simulink subsystem "hardware"  (R2024a)
settings: Solver=VariableStepAuto  StartTime=0.0  StopTime=10.0  RelTol=1e-3
model mask{RollOffset=0}
  mask prompts: RollOffset "Calibration Roll Offset"
undefined symbols (not defined in the file or in its folder): HS, IO291
libraries: speedgoatlib_IO691 x12, canmsglib x9, eeGeneralControl x6, aru_toolbox x4, speedgoatlib_IO291 x1
settings Model: Creator=Mechatronics  LastModifiedBy=user
settings ModelReferenceCC: EnableRefExpFcnMdlSchedulingChecks=on
settings RTWCC: GPUComputeCapability=3.5

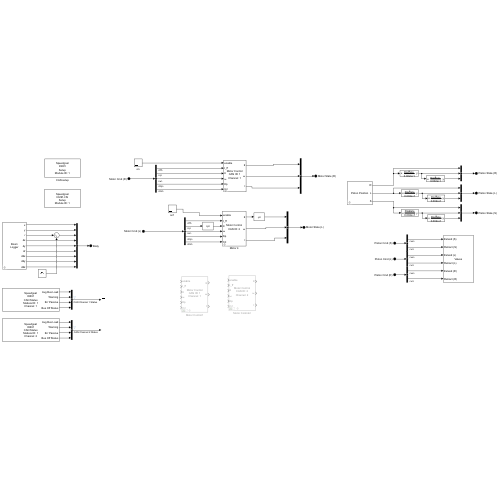
[thumbnail: Simulink's stored preview of the top-level diagram]
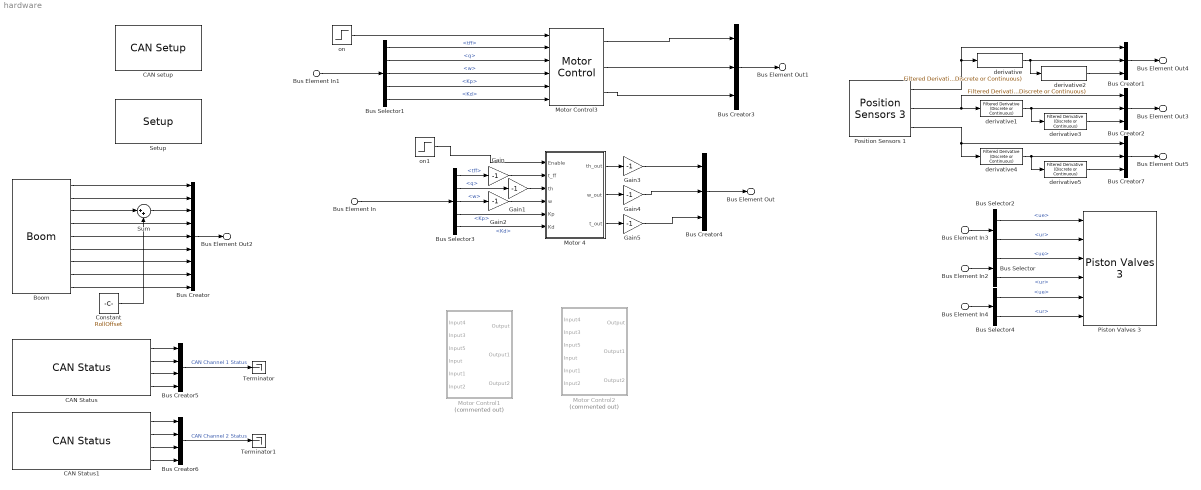
== system hardware ==
  Bus Element In : Inport  PortName=Motor Cmd (R)
  Bus Element In4 : Inport  Port=2  PortName=Piston Cmd (R)
  Bus Element In1 : Inport  Port=3  PortName=Motor Cmd (L)
  Bus Element In2 : Inport  Port=4  PortName=Piston Cmd (L)
  Bus Element In3 : Inport  Port=5  PortName=Piston Cmd (S)
  Boom : aru_toolbox/Boom  ts=0.001
      link override Serial Read HW FIFO: pciSlot=-1  board=IO393-50k
      link override Serial Setup: pciSlot=-1  board=IO393-50k
      settings: SourceProductName=ARU Toolbox
  Bus Creator : BusCreator  Inputs=9  OutDataTypeStr=Bus: BodyState  NonVirtualBus=on
      settings: InheritFromInputs=off
  Bus Creator1 : BusCreator  Inputs=3  OutDataTypeStr=Bus: PistonState  NonVirtualBus=on
      settings: InheritFromInputs=off
  Bus Creator2 : BusCreator  Inputs=3  OutDataTypeStr=Bus: PistonState  NonVirtualBus=on
      settings: InheritFromInputs=off
  Bus Creator3 : BusCreator  Inputs=3  OutDataTypeStr=Bus: MotorState  NonVirtualBus=on
      settings: InheritFromInputs=off
  Bus Creator4 : BusCreator  Inputs=3  OutDataTypeStr=Bus: MotorState  NonVirtualBus=on
      settings: InheritFromInputs=off
  Bus Creator5 : BusCreator  Inputs=4  OutDataTypeStr=Bus: CAN  NonVirtualBus=on
      settings: InheritFromInputs=off
  Bus Creator6 : BusCreator  Inputs=4  OutDataTypeStr=Bus: CAN  NonVirtualBus=on
      settings: InheritFromInputs=off
  Bus Creator7 : BusCreator  Inputs=3  OutDataTypeStr=Bus: PistonState  NonVirtualBus=on
      settings: InheritFromInputs=off
  Bus Selector : BusSelector  OutputSignals=ue,ur
  Bus Selector1 : BusSelector  OutputSignals=tff,q,w,Kp,Kd
  Bus Selector2 : BusSelector  OutputSignals=ue,ur
  Bus Selector3 : BusSelector  OutputSignals=tff,q,w,Kp,Kd
  Bus Selector4 : BusSelector  OutputSignals=ue,ur
  CAN Status : speedgoatlib_IO691/Legacy/CAN Status  moduleId=1  sampleTime=0.001  channel=1  busRecovery=Auto  arrayOutput=off  controllerCpuLoad=off  controllerLiveCount=off  initModeAct=off  avgBusLoad=on  receiving=off  RxQueueEmpty=off  dataOverrunRcv=off  rxBufferLevel=off  txPending=off  dataOverrunTx=off  txBufferLevel=off  errWarnLimit=on  errPassLimit=on  errBusOff=on  busRecoveryCounter=off  busCouplingErr=off  transceiverErr=off  opMode=off  brp=off  timeSegment1=off  timeSegment2=off  synchronisationJumpWidth=off  dataTSEG1=off  dataTSEG2=off  dataSJW=off  moduleType=691  qtyStatBlk=1  ptIdx=0  isFDMod=0
      settings: SourceProductName=IO691
  CAN Status1 : speedgoatlib_IO691/Legacy/CAN Status  moduleId=1  sampleTime=0.001  channel=2  busRecovery=Auto  arrayOutput=off  controllerCpuLoad=off  controllerLiveCount=off  initModeAct=off  avgBusLoad=on  receiving=off  RxQueueEmpty=off  dataOverrunRcv=off  rxBufferLevel=off  txPending=off  dataOverrunTx=off  txBufferLevel=off  errWarnLimit=on  errPassLimit=on  errBusOff=on  busRecoveryCounter=off  busCouplingErr=off  transceiverErr=off  opMode=off  brp=off  timeSegment1=off  timeSegment2=off  synchronisationJumpWidth=off  dataTSEG1=off  dataTSEG2=off  dataSJW=off  moduleType=691  qtyStatBlk=1  ptIdx=0  isFDMod=0
      settings: SourceProductName=IO691
  CAN setup : speedgoatlib_IO691/Legacy/CAN Setup   moduletype=IO691  id=1  pciSlot=-1  chn1=CAN (HS)  chn2=CAN (HS)  chn3=Disabled  chn4=Disabled  initStruct=[]  termStruct=[struct('Channel',1,'Protocol','CAN','BRS',0,'Type','Standard','Identifier',1,'Data',[255, 255, 255, 255, 255, 255, 255, 253],'Pause',0.001), struct('Channel',2,'Protocol','CAN','BRS',0,'Type','Standard','Identifier',2,'Data',[255, 255, 255, 255, 255, 255, 255, 253],'Pause',0.001)]  ArbitrationbdrChn1=1.0 MBaud  ArbitrationManbdrChn1=[2,8,31,8]  FdbdrChn1=1.0 MBaud  FdManbdrChn1=[2,8,31,8]  ArbitrationbdrChn2=1.0 MBaud  ArbitrationManbdrChn2=[2,8,31,8]  FdbdrChn2=1.0 MBaud  FdManbdrChn2=[2,8,31,8]  ArbitrationbdrChn3=1.0 MBaud  ArbitrationManbdrChn3=[2,8,31,8]  FdbdrChn3=5.0 MBaud  FdManbdrChn3=[2,2,5,2]  ArbitrationbdrChn4=1.0 MBaud  ArbitrationManbdrChn4=[2,8,31,8]  FdbdrChn4=5.0 MBaud  FdManbdrChn4=[2,2,5,2]  moduleInitValues=[691 1 -1 -1]
      settings: SourceProductName=IO691
  Constant : Constant  Value=RollOffset
  Gain{,1..5} (6 alike) : Gain  Gain=-1
  Motor 4 : Subsystem  mask{CAN_ID=2, channel=1}
      mask prompts: CAN_ID "CAN ID"
      mask init:
      | if exist("CAN_ID", "var")
      |         if CAN_ID == 1
      |             channel = 1;
      |             % set_param([gcb '/Enter Motor Mode/CAN Write Command'],'channel',sprintf('%d',1));
      |             % set_param([gcb '/CAN Write/CAN Write Command'],'channel',sprintf('%d',1));
      |             % set_param([gcb '/CAN Read/CAN Read Command'],'channel',sprintf('%d',1));
      |         end
      |         if CAN_ID == 2
      |             channel = 2;
      |             % set_param([gcb '/Enter Motor Mode/CAN Write Command'],'channel',sprintf('%d',2));
      |             % set_param([gcb '/CAN Write/CAN Write Command'],'channel',sprintf('%d',2));
      |             % set_param([gcb '/CAN Read/CAN Read Command'],'channel',sprintf('%d',2));
      |         end
      |     end
      mask TypeOptions channel: 1 | 2
      mask Display:
      | fprintf('Motor Control\nCAN ID: %c\n', get_param(gcb,'CAN_ID'));
      | port_label('input',1,'enable');
      | port_label('input',2,'t_ff');
      | port_label('input',3,'θ');
      | port_label('input',4,'ω');
      | port_label('input',5,'Kp');
      | port_label('input',6,'Kd');
      | port_label('output',1,'θ');
      | port_label('output',2,'ω');
      | port_label('output',3,'t');
  Motor Control1 : Subsystem  Commented=on  AncestorBlock=aru_toolbox/Motor Control  mask(Motor Control){id=1, channel=1, offset=-pi}
      mask prompts: offset "Position Offset (rad)"
      mask help: Generic control block for motors running Ben Katz's motor control firmware. (https://github.com/bgkatz/motorcontrol)
      mask TypeOptions channel: 1 | 2
      mask DialogControl ParameterGroupVar Prompt: CAN
      mask DialogControl Container4 Prompt: Control
      mask Display:
      | fprintf('Motor Control\nCAN ID: %c\nChannel: %c\n', get_param(gcb,'id'), get_param(gcb,'channel'));
      | port_label('input',1,'enable');
      | port_label('input',2,'t_ff');
      | port_label('input',3,'θ');
      | port_label('input',4,'ω');
      | port_label('input',5,'Kp');
      | port_label('input',6,'Kd');
      | port_label('output',1,'θ');
      | port_label('output',2,'ω');
      | port_label('output',3,'t');
  Motor Control2 : Subsystem  Commented=on  AncestorBlock=aru_toolbox/Motor Control  mask(Motor Control){id=2, channel=2, offset=0}
      mask prompts: offset "Position Offset (rad)"
      mask help: Generic control block for motors running Ben Katz's motor control firmware. (https://github.com/bgkatz/motorcontrol)
      mask TypeOptions channel: 1 | 2
      mask DialogControl ParameterGroupVar Prompt: CAN
      mask DialogControl Container4 Prompt: Control
      mask Display:
      | fprintf('Motor Control\nCAN ID: %c\nChannel: %c\n', get_param(gcb,'id'), get_param(gcb,'channel'));
      | port_label('input',1,'enable');
      | port_label('input',2,'t_ff');
      | port_label('input',3,'θ');
      | port_label('input',4,'ω');
      | port_label('input',5,'Kp');
      | port_label('input',6,'Kd');
      | port_label('output',1,'θ');
      | port_label('output',2,'ω');
      | port_label('output',3,'t');
  Motor Control3 : aru_toolbox/Motor Control  id=1  channel=1  offset=0
      settings: SourceProductName=ARU Toolbox
  Piston Valves 3 : aru_toolbox/Piston Valves 3  SystemSampleTime=-1  VariantActivationTime=update diagram  AllowFlexibleInterface=on  Latency=0  AutoFrameSizeCalculation=off
      settings: SourceProductName=ARU Toolbox
  Position Sensors 1 : aru_toolbox/Position Sensors 3  stroke1=0.07  min_r=803  max_r=3724  stroke2=0.07  min_l=743  max_l=3646  stroke3=0.2  min_s=741  max_s=3392
      settings: SourceProductName=ARU Toolbox
  "Setup " : speedgoatlib_IO291/Setup   parInternalModuleId=1  parPciSlot=-1  parModuleId=1  parModuleType=IO291-HS  parTtlDoChannels=[]  parTtlDoInitValues=1  parTtlDoReset=1  parTtlDiChannels=[1 2 3 4 5]  parIsolDiChannels=[]  parFetDoChannels=[1 2 3 4 5 6]  parFetDoInitValues=0  parFetDoReset=1
      settings: SourceProductName=IO291
  Sum : Sum  Inputs=|++
  Terminator : Terminator
  Terminator1 : Terminator
  derivative{,1..5} (6 alike) : eeGeneralControl/Filtered Derivative (Discrete or Continuous)  K=1  T=0.002  B=inf  A=-inf  minRatio=2  init_option=Inherited from block input  x0=0  Ts=0.001
  on : Step  SampleTime=0
  on1 : Step  Time=2  SampleTime=0
  Bus Element Out : Outport  PortName=Motor State (R)
  Bus Element Out4 : Outport  Port=2  PortName=Piston State (R)
  Bus Element Out1 : Outport  Port=3  PortName=Motor State (L)
  Bus Element Out3 : Outport  Port=4  PortName=Piston State (L)
  Bus Element Out2 : Outport  Port=5  PortName=Body
  Bus Element Out5 : Outport  Port=6  PortName=Piston State (S)
  wires:
  Bus Selector1/1 -> Motor Control3/2  "<tff>"
  Bus Creator5/1 -> Terminator/1  "CAN Channel 1 Status"
  derivative2/1 -> Bus Creator1/3
  Bus Selector/1 -> Piston Valves 3/3  "<ue>"
  Bus Element In1/1 -> Bus Selector1/1
  Bus Selector1/4 -> Motor Control3/5  "<Kp>"
  Bus Selector/2 -> Piston Valves 3/4  "<ur>"
  Bus Selector3/4 -> Motor 4/5(Kp)  "<Kp>"
  Bus Selector3/2 -> Gain1/1  "<q>"
  Bus Selector2/2 -> Piston Valves 3/2  "<ur>"
  Bus Creator6/1 -> Terminator1/1  "CAN Channel 2 Status"
  CAN Status1/3 -> Bus Creator6/3
  on1/1 -> Motor 4/1(Enable)
  Bus Selector2/1 -> Piston Valves 3/1  "<ue>"
  Bus Element In3/1 -> Bus Selector2/1
  Bus Selector1/3 -> Motor Control3/4  "<w>"
  CAN Status1/4 -> Bus Creator6/4
  Bus Selector3/1 -> Gain/1  "<tff>"
  Boom/1 -> Bus Creator/1
  Boom/3 -> Sum/1
  Bus Element In2/1 -> Bus Selector/1
  CAN Status/3 -> Bus Creator5/3
  Bus Creator1/1 -> Bus Element Out4/1
  Boom/7 -> Bus Creator/7
  Boom/5 -> Bus Creator/5
  Boom/6 -> Bus Creator/6
  Bus Creator/1 -> Bus Element Out2/1
  Bus Selector3/5 -> Motor 4/6(Kd)  "<Kd>"
  Boom/8 -> Bus Creator/8
  Boom/4 -> Bus Creator/4
  Bus Selector1/2 -> Motor Control3/3  "<q>"
  derivative/1 -> derivative2/1, Bus Creator1/2
  derivative3/1 -> Bus Creator2/3
  CAN Status/4 -> Bus Creator5/4
  Bus Selector3/3 -> Gain2/1  "<w>"
  derivative1/1 -> derivative3/1, Bus Creator2/2
  Boom/2 -> Bus Creator/2
  CAN Status1/2 -> Bus Creator6/2
  Position Sensors 1/2 -> derivative1/1, Bus Creator2/1
  Bus Element In/1 -> Bus Selector3/1
  Bus Selector1/5 -> Motor Control3/6  "<Kd>"
  Constant/1 -> Sum/2
  CAN Status/1 -> Bus Creator5/1
  Boom/9 -> Bus Creator/9
  Position Sensors 1/1 -> Bus Creator1/1, derivative/1
  Sum/1 -> Bus Creator/3
  on/1 -> Motor Control3/1
  CAN Status1/1 -> Bus Creator6/1
  Bus Creator2/1 -> Bus Element Out3/1
  CAN Status/2 -> Bus Creator5/2
  Motor 4/2(w_out) -> Gain4/1
  Motor 4/3(t_out) -> Gain5/1
  Bus Selector4/2 -> Piston Valves 3/6  "<ur>"
  Bus Selector4/1 -> Piston Valves 3/5  "<ue>"
  Bus Element In4/1 -> Bus Selector4/1
  derivative4/1 -> derivative5/1, Bus Creator7/2
  Bus Creator7/1 -> Bus Element Out5/1
  derivative5/1 -> Bus Creator7/3
  Position Sensors 1/3 -> Bus Creator7/1, derivative4/1
  Motor Control3/1 -> Bus Creator3/1
  Motor Control3/2 -> Bus Creator3/2
  Motor Control3/3 -> Bus Creator3/3
  Motor 4/1(th_out) -> Gain3/1
  Bus Creator4/1 -> Bus Element Out/1
  Bus Creator3/1 -> Bus Element Out1/1
  Gain/1 -> Motor 4/2(t_ff)
  Gain1/1 -> Motor 4/3(th)
  Gain2/1 -> Motor 4/4(w)
  Gain3/1 -> Bus Creator4/1
  Gain4/1 -> Bus Creator4/2
  Gain5/1 -> Bus Creator4/3

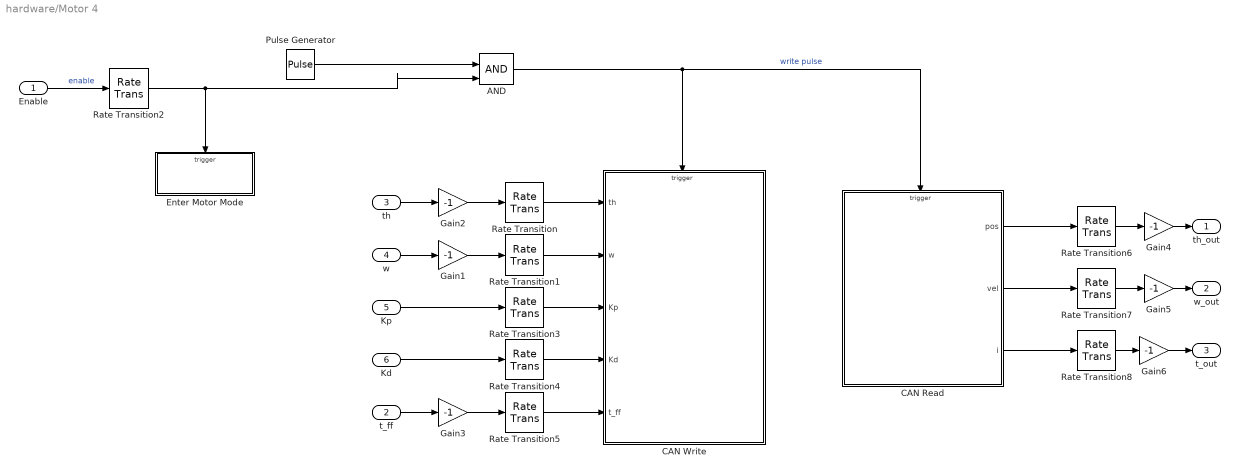
== system hardware/Motor 4 ==
  Enable : Inport
  t_ff : Inport  Port=2
  th : Inport  Port=3
  w : Inport  Port=4
  Kp : Inport  Port=5
  Kd : Inport  Port=6
  AND : Logic  IconShape=distinctive  AllPortsSameDT=off  OutDataTypeStr=boolean
  CAN Read : Subsystem  LoadFcn=set_param([gcb '/CAN Read Command'], 'channel', sprintf('%d', channel));  TreatAsAtomicUnit=on
  CAN Write : Subsystem  LoadFcn=set_param([gcb '/CAN Write Command'], 'channel', sprintf('%d', channel));
  Enter Motor Mode : Subsystem  LoadFcn=set_param([gcb '/CAN Write Command'], 'channel', sprintf('%d', channel));  TreatAsAtomicUnit=on
  Gain{1..6} (6 alike) : Gain  Gain=-1
  Pulse Generator : DiscretePulseGenerator  PulseType=Time based  Period=1/1000  PulseWidth=50
  Rate Transition{,1..8} (9 alike) : RateTransition
  th_out : Outport
  w_out : Outport  Port=2
  t_out : Outport  Port=3
  wires:
  Gain6/1 -> t_out/1
  Gain5/1 -> w_out/1
  Gain4/1 -> th_out/1
  Gain3/1 -> Rate Transition5/1
  Gain1/1 -> Rate Transition1/1
  Gain2/1 -> Rate Transition/1
  Rate Transition2/1 -> Enter Motor Mode/Trigger, AND/2
  Pulse Generator/1 -> AND/1
  AND/1 -> CAN Read/Trigger, CAN Write/Trigger  "write pulse"
  Enable/1 -> Rate Transition2/1  "enable"
  Rate Transition5/1 -> CAN Write/5(t_ff)
  Rate Transition/1 -> CAN Write/1(th)
  th/1 -> Gain2/1
  t_ff/1 -> Gain3/1
  Kd/1 -> Rate Transition4/1
  Kp/1 -> Rate Transition3/1
  w/1 -> Gain1/1
  Rate Transition1/1 -> CAN Write/2(w)
  Rate Transition3/1 -> CAN Write/3(Kp)
  Rate Transition4/1 -> CAN Write/4(Kd)
  CAN Read/1(pos) -> Rate Transition6/1
  CAN Read/2(vel) -> Rate Transition7/1
  CAN Read/3(i) -> Rate Transition8/1
  Rate Transition6/1 -> Gain4/1
  Rate Transition8/1 -> Gain6/1
  Rate Transition7/1 -> Gain5/1

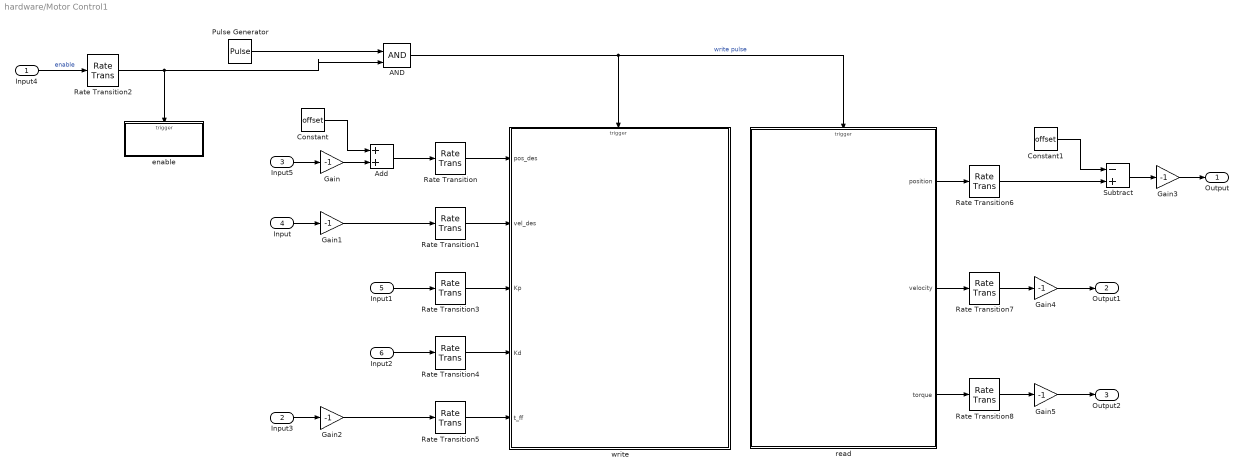
== system hardware/Motor Control1 ==
  Input4 : Inport
  Input3 : Inport  Port=2
  Input5 : Inport  Port=3
  Input : Inport  Port=4
  Input1 : Inport  Port=5
  Input2 : Inport  Port=6
  AND : Logic  IconShape=distinctive  AllPortsSameDT=off  OutDataTypeStr=boolean
  Add : Sum
  Constant : Constant  Value=offset
  Constant1 : Constant  Value=offset
  Gain{,1..5} (6 alike) : Gain  Gain=-1
  Pulse Generator : DiscretePulseGenerator  PulseType=Time based  Period=0.001  PulseWidth=50
  Rate Transition{,1..8} (9 alike) : RateTransition
  Subtract : Sum  Inputs=-+
  enable : Subsystem  TreatAsAtomicUnit=on
  read : Subsystem  TreatAsAtomicUnit=on
  write : Subsystem  TreatAsAtomicUnit=on
  Output : Outport
  Output1 : Outport  Port=2
  Output2 : Outport  Port=3
  wires:
  Gain5/1 -> Output2/1
  Gain4/1 -> Output1/1
  Gain3/1 -> Output/1
  Gain2/1 -> Rate Transition5/1
  Gain1/1 -> Rate Transition1/1
  Gain/1 -> Add/2
  Constant1/1 -> Subtract/1
  Rate Transition6/1 -> Subtract/2
  Subtract/1 -> Gain3/1
  Constant/1 -> Add/1
  Add/1 -> Rate Transition/1
  Input5/1 -> Gain/1
  Rate Transition8/1 -> Gain5/1
  Rate Transition7/1 -> Gain4/1
  Rate Transition5/1 -> write/5(t_ff)
  Rate Transition4/1 -> write/4(Kd)
  Rate Transition3/1 -> write/3(Kp)
  Rate Transition2/1 -> AND/2, enable/Trigger
  Rate Transition1/1 -> write/2(vel_des)
  Rate Transition/1 -> write/1(pos_des)
  read/1(position) -> Rate Transition6/1
  Input4/1 -> Rate Transition2/1  "enable"
  AND/1 -> write/Trigger, read/Trigger  "write pulse"
  Pulse Generator/1 -> AND/1
  Input/1 -> Gain1/1
  read/3(torque) -> Rate Transition8/1
  read/2(velocity) -> Rate Transition7/1
  Input2/1 -> Rate Transition4/1
  Input3/1 -> Gain2/1
  Input1/1 -> Rate Transition3/1

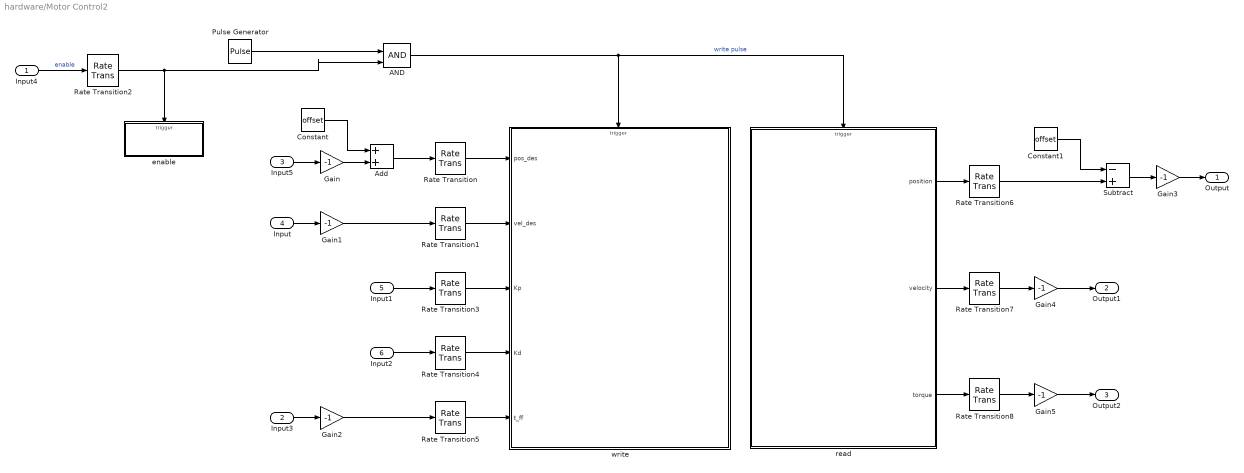
== system hardware/Motor Control2 ==
  Input4 : Inport
  Input3 : Inport  Port=2
  Input5 : Inport  Port=3
  Input : Inport  Port=4
  Input1 : Inport  Port=5
  Input2 : Inport  Port=6
  AND : Logic  IconShape=distinctive  AllPortsSameDT=off  OutDataTypeStr=boolean
  Add : Sum
  Constant : Constant  Value=offset
  Constant1 : Constant  Value=offset
  Gain{,1..5} (6 alike) : Gain  Gain=-1
  Pulse Generator : DiscretePulseGenerator  PulseType=Time based  Period=0.001  PulseWidth=50
  Rate Transition{,1..8} (9 alike) : RateTransition
  Subtract : Sum  Inputs=-+
  enable : Subsystem  TreatAsAtomicUnit=on
  read : Subsystem  TreatAsAtomicUnit=on
  write : Subsystem  TreatAsAtomicUnit=on
  Output : Outport
  Output1 : Outport  Port=2
  Output2 : Outport  Port=3
  wires:
  Input1/1 -> Rate Transition3/1
  Input3/1 -> Gain2/1
  Input2/1 -> Rate Transition4/1
  read/2(velocity) -> Rate Transition7/1
  read/3(torque) -> Rate Transition8/1
  Input/1 -> Gain1/1
  Pulse Generator/1 -> AND/1
  AND/1 -> read/Trigger, write/Trigger  "write pulse"
  Input4/1 -> Rate Transition2/1  "enable"
  read/1(position) -> Rate Transition6/1
  Rate Transition/1 -> write/1(pos_des)
  Rate Transition1/1 -> write/2(vel_des)
  Rate Transition2/1 -> enable/Trigger, AND/2
  Rate Transition3/1 -> write/3(Kp)
  Rate Transition4/1 -> write/4(Kd)
  Rate Transition5/1 -> write/5(t_ff)
  Rate Transition7/1 -> Gain4/1
  Rate Transition8/1 -> Gain5/1
  Input5/1 -> Gain/1
  Add/1 -> Rate Transition/1
  Constant/1 -> Add/1
  Subtract/1 -> Gain3/1
  Rate Transition6/1 -> Subtract/2
  Constant1/1 -> Subtract/1
  Gain/1 -> Add/2
  Gain1/1 -> Rate Transition1/1
  Gain2/1 -> Rate Transition5/1
  Gain3/1 -> Output/1
  Gain4/1 -> Output1/1
  Gain5/1 -> Output2/1

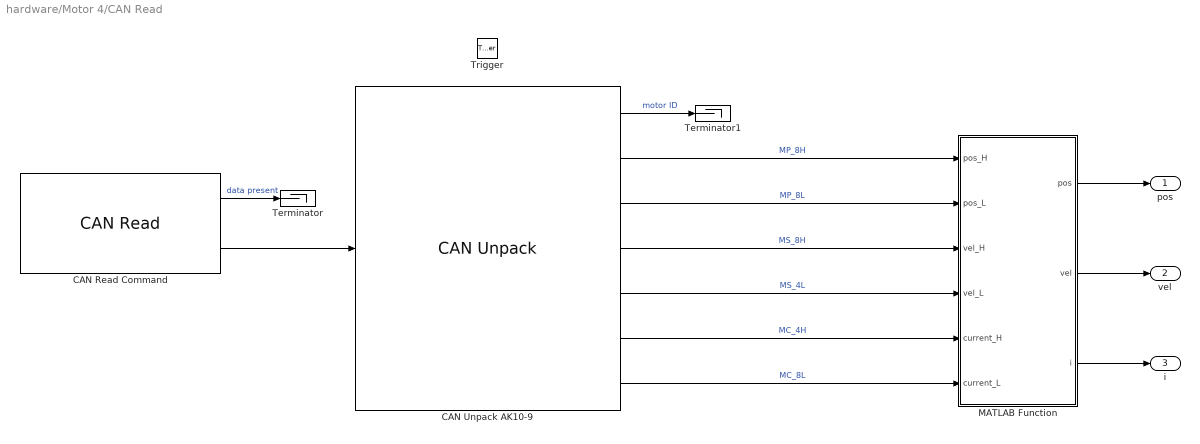
== system hardware/Motor 4/CAN Read ==
  Trigger : TriggerPort  TriggerType=either  VariantControl=(inherit)  PortDimensions=1
  CAN Read Command : speedgoatlib_IO691/Legacy/CAN Read  id=1  ts=-1  channel=2  messageType=CAN  canType=CAN (HS)  BusOutput=off  initValues=[691 1 -1 1 1 1 0]
      settings: SourceProductName=IO691
  CAN Unpack AK10-9 : canmsglib/CAN Unpack  MsgList=(none)  MsgName=CAN Msg  MsgIDType=Standard (11-bit identifier)  MsgIdentifier=0  MsgLength=8  SignalInfo={ 'Drive ID', '0', '8', 'LE', 'unsigned', 'Standard', '0', '1', '0', '-Inf', 'Inf'; 'Motor position 8-H', '8', '8', 'LE', 'unsigned', 'Standard', '0', '1', '0', '-Inf', 'Inf'; 'Motor position 8-L', '16', '8', 'LE', 'unsigned', 'Standard', '0', '1', '0', '-Inf', 'Inf'; 'Motor speed 8-H', '24', '8', 'LE', 'unsigned', 'Standard', '0', '1', '0', '-Inf', 'Inf'; 'Motor speed 4-L', '36', '4', 'LE', 'unsigned', 'Standard', '0', '1', '0', '-Inf', 'Inf'; 'Current 4-H', '32', '4', 'LE', 'unsigned', 'Standard', '0', '1', '0', '-Inf', 'Inf'; 'Current 8-L', '40', '8', 'LE', 'unsigned', 'Standard', '0', '1', '0', '-Inf', 'Inf' }  IDPort=off  TimestampPort=off  ErrorPort=off  RemotePort=off  LengthPort=off  StatusPort=off  ApplyMinMax=off
  MATLAB Function : MATLAB Function  TreatAsAtomicUnit=on
  Terminator : Terminator
  Terminator1 : Terminator
  pos : Outport
  vel : Outport  Port=2
  i : Outport  Port=3
  wires:
  CAN Unpack AK10-9/4 -> MATLAB Function/3(vel_H)  "MS_8H"
  MATLAB Function/1(pos) -> pos/1
  CAN Unpack AK10-9/7 -> MATLAB Function/6(current_L)  "MC_8L"
  CAN Unpack AK10-9/6 -> MATLAB Function/5(current_H)  "MC_4H"
  CAN Unpack AK10-9/2 -> MATLAB Function/1(pos_H)  "MP_8H"
  CAN Unpack AK10-9/1 -> Terminator1/1  "motor ID"
  CAN Unpack AK10-9/5 -> MATLAB Function/4(vel_L)  "MS_4L"
  CAN Unpack AK10-9/3 -> MATLAB Function/2(pos_L)  "MP_8L"
  MATLAB Function/3(i) -> i/1
  MATLAB Function/2(vel) -> vel/1
  CAN Read Command/1 -> Terminator/1  "data present"
  CAN Read Command/2 -> CAN Unpack AK10-9/1

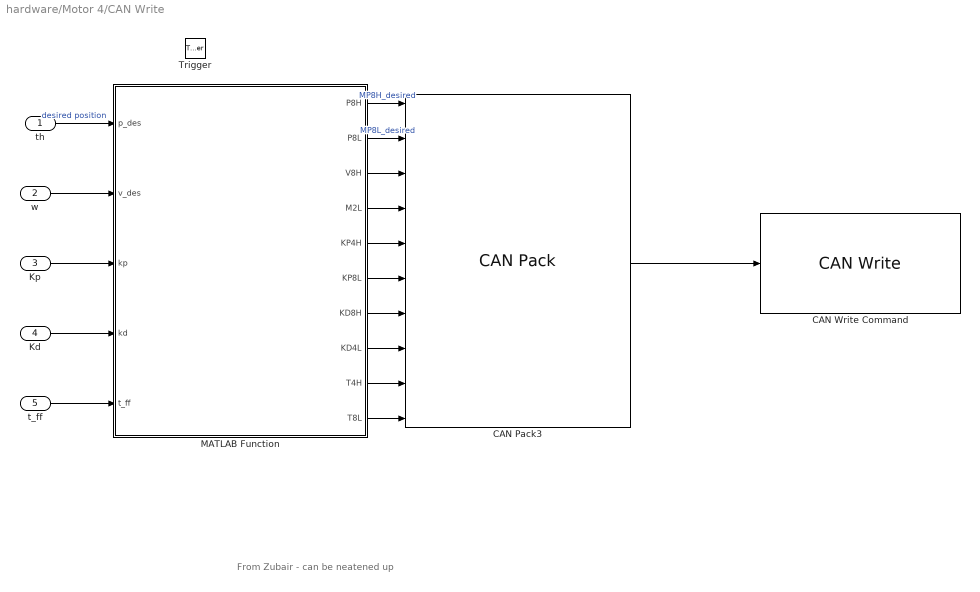
== system hardware/Motor 4/CAN Write ==
  note: From Zubair - can be neatened up
  th : Inport
  w : Inport  Port=2
  Kp : Inport  Port=3
  Kd : Inport  Port=4
  t_ff : Inport  Port=5
  Trigger : TriggerPort  VariantControl=Variant
  CAN Pack3 : canmsglib/CAN Pack  MsgList=(none)  MsgName=MotorControl  MsgIDType=Standard (11-bit identifier)  MsgIdentifier=CAN_ID  MsgLength=8  Remote=off  ApplyMinMax=off  BusOutput=off  SignalInfo={ 'Motor postition 8-H', '0', '8', 'LE', 'unsigned', 'Standard', '0', '1', '0', '-Inf', 'Inf'; 'Motor position 8-L', '8', '8', 'LE', 'unsigned', 'Standard', '0', '1', '0', '-Inf', 'Inf'; 'Motor speed 8-H', '16', '8', 'LE', 'unsigned', 'Standard', '0', '1', '0', '-Inf', 'Inf'; 'Motor speed 4-L', '28', '4', 'LE', 'unsigned', 'Standard', '0', '1', '0', '-Inf', 'Inf'; 'KP 4-H', '24', '4', 'LE', 'unsigned', 'Standard', '0', '1', '0', '-Inf', 'Inf'; 'KP 8-L', '32', '8', 'LE', 'unsigned', 'Standard', '0', '1', '0', '-Inf', 'Inf'; 'KD 8-H', '40', '8', 'LE', 'unsigned', 'Standard', '0', '1', '0', '-Inf', 'Inf'; 'KD 4-L', '52', '4', 'LE', 'unsigned', 'Standard', '0', '1', '0', '-Inf', 'Inf'; 'Current 4-H', '48', '4', 'LE', 'unsigned', 'Standard', '0', '1', '0', '-Inf', 'Inf'; 'Current 8-L', '56', '8', 'LE', 'unsigned', 'Standard', '0', '1', '0', '-Inf', 'Inf' }
      settings: DataFormat=manually specified signals
  CAN Write Command : speedgoatlib_IO691/Legacy/CAN Write  id=1  ts=-1  channel=2  messageType=CAN  BusInput=off  enableStatusPort=off  canType=CAN (HS)  initValues=[691 1 -1 1 1 1 0 0]
      settings: SourceProductName=IO691
  MATLAB Function : MATLAB Function  TreatAsAtomicUnit=on
  wires:
  CAN Pack3/1 -> CAN Write Command/1
  MATLAB Function/1(P8H) -> CAN Pack3/1  "MP8H_desired"
  MATLAB Function/7(KD8H) -> CAN Pack3/7
  Kp/1 -> MATLAB Function/3(kp)
  MATLAB Function/9(T4H) -> CAN Pack3/9
  w/1 -> MATLAB Function/2(v_des)
  Kd/1 -> MATLAB Function/4(kd)
  MATLAB Function/6(KP8L) -> CAN Pack3/6
  th/1 -> MATLAB Function/1(p_des)  "desired position"
  MATLAB Function/10(T8L) -> CAN Pack3/10
  MATLAB Function/2(P8L) -> CAN Pack3/2  "MP8L_desired"
  MATLAB Function/5(KP4H) -> CAN Pack3/5
  MATLAB Function/3(V8H) -> CAN Pack3/3
  t_ff/1 -> MATLAB Function/5(t_ff)
  MATLAB Function/8(KD4L) -> CAN Pack3/8
  MATLAB Function/4(M2L) -> CAN Pack3/4

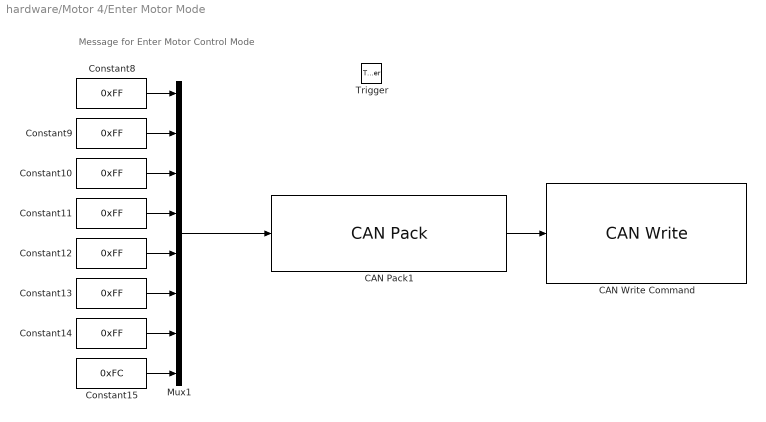
== system hardware/Motor 4/Enter Motor Mode ==
  note: Message for Enter Motor Control Mode
  Trigger : TriggerPort  VariantControl=(inherit)
  CAN Pack1 : canmsglib/CAN Pack  MsgList=(none)  MsgName=CAN Msg  MsgIDType=Standard (11-bit identifier)  MsgIdentifier=CAN_ID  MsgLength=8  Remote=off  ApplyMinMax=off  BusOutput=off  SignalInfo={ 'Motor postition 8-H', '0', '8', 'LE', 'unsigned', 'Standard', '0', '1', '0', '-Inf', 'Inf'; 'Motor position 8-L', '8', '8', 'LE', 'unsigned', 'Standard', '0', '1', '0', '-Inf', 'Inf'; 'Motor seed 8-H', '16', '8', 'LE', 'unsigned', 'Standard', '0', '1', '0', '-Inf', 'Inf'; 'Motor speed 4-L', '28', '4', 'LE', 'unsigned', 'Standard', '0', '1', '0', '-Inf', 'Inf'; 'KP 4-H', '24', '4', 'LE', 'unsigned', 'Standard', '0', '1', '0', '-Inf', 'Inf'; 'KP 8-L', '32', '8', 'LE', 'unsigned', 'Standard', '0', '1', '0', '-Inf', 'Inf'; 'KP 8-H', '40', '8', 'LE', 'unsigned', 'Standard', '0', '1', '0', '-Inf', 'Inf'; 'KD 4-L', '52', '4', 'LE', 'unsigned', 'Standard', '0', '1', '0', '-Inf', 'Inf'; 'Current 4-H', '48', '4', 'LE', 'unsigned', 'Standard', '0', '1', '0', '-Inf', 'Inf'; 'Current 8-L', '56', '8', 'LE', 'unsigned', 'Standard', '0', '1', '0', '-Inf', 'Inf' }
      settings: DataFormat=raw data
  CAN Write Command : speedgoatlib_IO691/Legacy/CAN Write  id=1  ts=-1  channel=2  messageType=CAN  BusInput=off  enableStatusPort=off  canType=CAN (HS)  initValues=[691 1 -1 1 1 1 0 0]
      settings: SourceProductName=IO691
  Constant{8..14} (7 alike) : Constant  Value=0xFF  OutDataTypeStr=uint8  SampleTime=-1
  Constant15 : Constant  Value=0xFC  OutDataTypeStr=uint8  SampleTime=-1
  Mux1 : Mux  Inputs=8
  wires:
  Constant10/1 -> Mux1/3
  Constant13/1 -> Mux1/6
  Mux1/1 -> CAN Pack1/1
  Constant14/1 -> Mux1/7
  Constant9/1 -> Mux1/2
  Constant15/1 -> Mux1/8
  Constant11/1 -> Mux1/4
  Constant8/1 -> Mux1/1
  Constant12/1 -> Mux1/5
  CAN Pack1/1 -> CAN Write Command/1

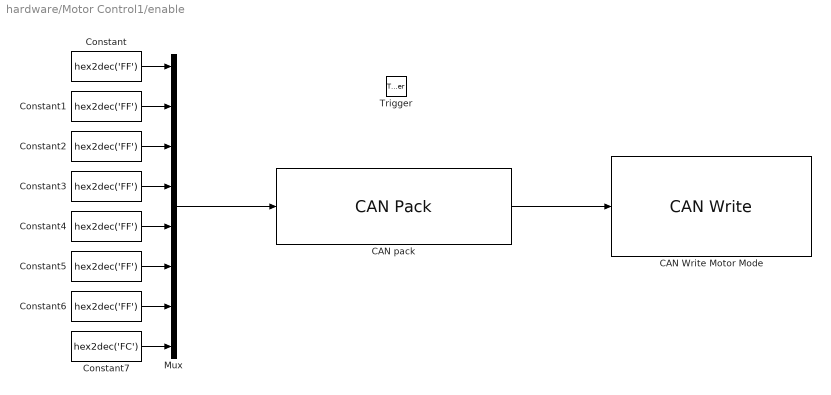
== system hardware/Motor Control1/enable ==
  Trigger : TriggerPort  VariantControl=Variant
  CAN Write Motor Mode : speedgoatlib_IO691/Legacy/CAN Write  id=1  ts=-1  channel=1  messageType=CAN  BusInput=off  enableStatusPort=off  canType=CAN (HS)  initValues=[691 1 -1 0 1 1 0 0]
      settings: SourceProductName=IO691
  CAN pack : canmsglib/CAN Pack  MsgList=(none)  MsgName=enable  MsgIDType=Standard (11-bit identifier)  MsgIdentifier=id  MsgLength=8  Remote=off  ApplyMinMax=off  BusOutput=off  SignalInfo={ 'Motor postition 8-H', '0', '8', 'LE', 'unsigned', 'Standard', '0', '1', '0', '-Inf', 'Inf'; 'Motor position 8-L', '8', '8', 'LE', 'unsigned', 'Standard', '0', '1', '0', '-Inf', 'Inf'; 'Motor seed 8-H', '16', '8', 'LE', 'unsigned', 'Standard', '0', '1', '0', '-Inf', 'Inf'; 'Motor speed 4-L', '28', '4', 'LE', 'unsigned', 'Standard', '0', '1', '0', '-Inf', 'Inf'; 'KP 4-H', '24', '4', 'LE', 'unsigned', 'Standard', '0', '1', '0', '-Inf', 'Inf'; 'KP 8-L', '32', '8', 'LE', 'unsigned', 'Standard', '0', '1', '0', '-Inf', 'Inf'; 'KP 8-H', '40', '8', 'LE', 'unsigned', 'Standard', '0', '1', '0', '-Inf', 'Inf'; 'KD 4-L', '52', '4', 'LE', 'unsigned', 'Standard', '0', '1', '0', '-Inf', 'Inf'; 'Current 4-H', '48', '4', 'LE', 'unsigned', 'Standard', '0', '1', '0', '-Inf', 'Inf'; 'Current 8-L', '56', '8', 'LE', 'unsigned', 'Standard', '0', '1', '0', '-Inf', 'Inf' }
      settings: DataFormat=raw data
  Constant{,1..6} (7 alike) : Constant  Value=hex2dec('FF')  OutDataTypeStr=uint8  SampleTime=-1
  Constant7 : Constant  Value=hex2dec('FC')  OutDataTypeStr=uint8  SampleTime=-1
  Mux : Mux  Inputs=8
  wires:
  Constant6/1 -> Mux/7
  Constant/1 -> Mux/1
  Constant2/1 -> Mux/3
  Constant3/1 -> Mux/4
  Constant5/1 -> Mux/6
  Constant1/1 -> Mux/2
  Constant4/1 -> Mux/5
  Constant7/1 -> Mux/8
  Mux/1 -> CAN pack/1
  CAN pack/1 -> CAN Write Motor Mode/1

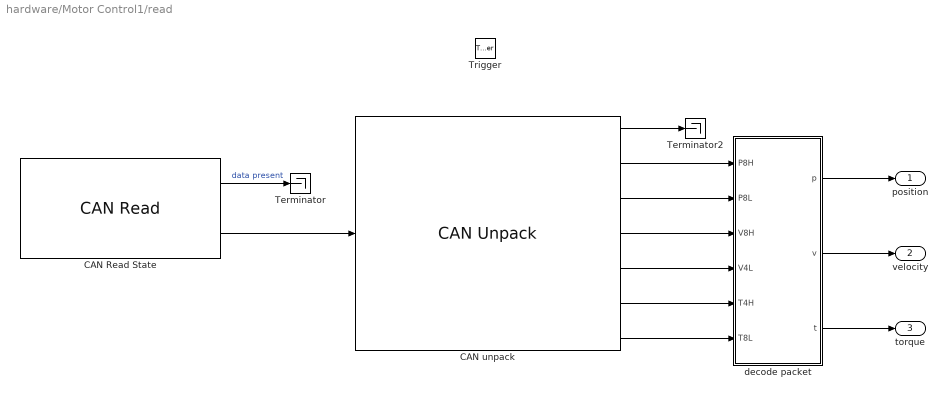
== system hardware/Motor Control1/read ==
  Trigger : TriggerPort  TriggerType=either  VariantControl=Variant
  CAN Read State : speedgoatlib_IO691/Legacy/CAN Read  id=1  ts=-1  channel=1  messageType=CAN  canType=CAN (HS)  BusOutput=off  initValues=[691 1 -1 0 1 1 0]
      settings: SourceProductName=IO691
  CAN unpack : canmsglib/CAN Unpack  MsgList=(none)  MsgName=CAN Msg  MsgIDType=Standard (11-bit identifier)  MsgIdentifier=0  MsgLength=6  SignalInfo={ 'ID', '0', '8', 'LE', 'unsigned', 'Standard', '0', '1', '0', '-Inf', 'Inf'; 'P8H', '8', '8', 'LE', 'unsigned', 'Standard', '0', '1', '0', '-Inf', 'Inf'; 'P8L', '16', '8', 'LE', 'unsigned', 'Standard', '0', '1', '0', '-Inf', 'Inf'; 'V8H', '24', '8', 'LE', 'unsigned', 'Standard', '0', '1', '0', '-Inf', 'Inf'; 'V4L', '36', '4', 'LE', 'unsigned', 'Standard', '0', '1', '0', '-Inf', 'Inf'; 'I4H', '32', '4', 'LE', 'unsigned', 'Standard', '0', '1', '0', '-Inf', 'Inf'; 'I8L', '40', '8', 'LE', 'unsigned', 'Standard', '0', '1', '0', '-Inf', 'Inf' }  IDPort=off  TimestampPort=off  ErrorPort=off  RemotePort=off  LengthPort=off  StatusPort=off  ApplyMinMax=off
  Terminator : Terminator
  Terminator2 : Terminator
  decode packet : MATLAB Function  TreatAsAtomicUnit=on
  position : Outport
  velocity : Outport  Port=2
  torque : Outport  Port=3
  wires:
  CAN Read State/1 -> Terminator/1  "data present"
  decode packet/3(t) -> torque/1
  decode packet/1(p) -> position/1
  decode packet/2(v) -> velocity/1
  CAN unpack/4 -> decode packet/3(V8H)
  CAN unpack/7 -> decode packet/6(T8L)
  CAN unpack/2 -> decode packet/1(P8H)
  CAN unpack/3 -> decode packet/2(P8L)
  CAN unpack/5 -> decode packet/4(V4L)
  CAN unpack/6 -> decode packet/5(T4H)
  CAN Read State/2 -> CAN unpack/1
  CAN unpack/1 -> Terminator2/1

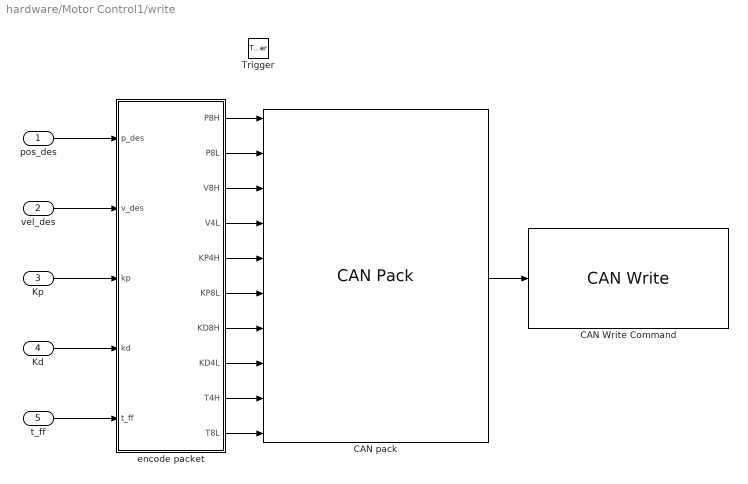
== system hardware/Motor Control1/write ==
  pos_des : Inport
  vel_des : Inport  Port=2
  Kp : Inport  Port=3
  Kd : Inport  Port=4
  t_ff : Inport  Port=5
  Trigger : TriggerPort  VariantControl=Variant
  CAN Write Command : speedgoatlib_IO691/Legacy/CAN Write  id=1  ts=-1  channel=1  messageType=CAN  BusInput=off  enableStatusPort=off  canType=CAN (HS)  initValues=[691 1 -1 0 1 1 0 0]
      settings: SourceProductName=IO691
  CAN pack : canmsglib/CAN Pack  MsgList=(none)  MsgName=MotorControl  MsgIDType=Standard (11-bit identifier)  MsgIdentifier=id  MsgLength=8  Remote=off  ApplyMinMax=off  BusOutput=off  SignalInfo={ 'P8H', '0', '8', 'LE', 'unsigned', 'Standard', '0', '1', '0', '-Inf', 'Inf'; 'P8L', '8', '8', 'LE', 'unsigned', 'Standard', '0', '1', '0', '-Inf', 'Inf'; 'V8H', '16', '8', 'LE', 'unsigned', 'Standard', '0', '1', '0', '-Inf', 'Inf'; 'V4L', '28', '4', 'LE', 'unsigned', 'Standard', '0', '1', '0', '-Inf', 'Inf'; 'KP4H', '24', '4', 'LE', 'unsigned', 'Standard', '0', '1', '0', '-Inf', 'Inf'; 'KP8L', '32', '8', 'LE', 'unsigned', 'Standard', '0', '1', '0', '-Inf', 'Inf'; 'KD8H', '40', '8', 'LE', 'unsigned', 'Standard', '0', '1', '0', '-Inf', 'Inf'; 'KD4L', '52', '4', 'LE', 'unsigned', 'Standard', '0', '1', '0', '-Inf', 'Inf'; 'T4H', '48', '4', 'LE', 'unsigned', 'Standard', '0', '1', '0', '-Inf', 'Inf'; 'T8L', '56', '8', 'LE', 'unsigned', 'Standard', '0', '1', '0', '-Inf', 'Inf' }
      settings: DataFormat=manually specified signals
  encode packet : MATLAB Function  TreatAsAtomicUnit=on
  wires:
  encode packet/10(T8L) -> CAN pack/10
  encode packet/3(V8H) -> CAN pack/3
  CAN pack/1 -> CAN Write Command/1
  encode packet/1(P8H) -> CAN pack/1
  encode packet/9(T4H) -> CAN pack/9
  encode packet/4(V4L) -> CAN pack/4
  encode packet/8(KD4L) -> CAN pack/8
  t_ff/1 -> encode packet/5(t_ff)
  Kd/1 -> encode packet/4(kd)
  encode packet/5(KP4H) -> CAN pack/5
  Kp/1 -> encode packet/3(kp)
  encode packet/2(P8L) -> CAN pack/2
  encode packet/7(KD8H) -> CAN pack/7
  encode packet/6(KP8L) -> CAN pack/6
  pos_des/1 -> encode packet/1(p_des)
  vel_des/1 -> encode packet/2(v_des)

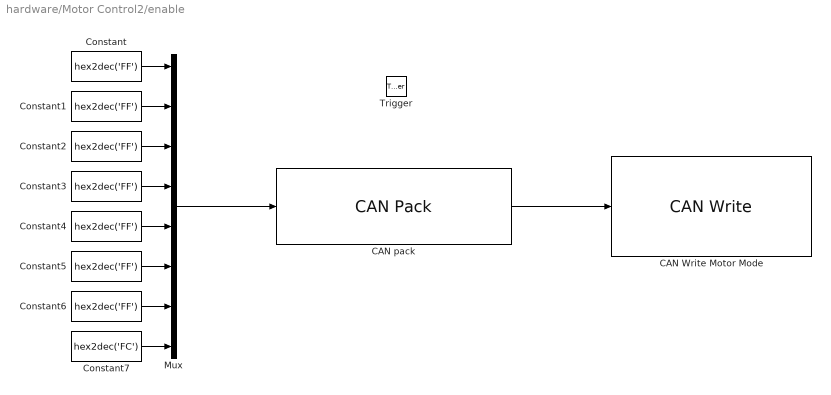
== system hardware/Motor Control2/enable ==
  Trigger : TriggerPort  VariantControl=Variant
  CAN Write Motor Mode : speedgoatlib_IO691/Legacy/CAN Write  id=1  ts=-1  channel=2  messageType=CAN  BusInput=off  enableStatusPort=off  canType=CAN (HS)  initValues=[691 1 -1 1 1 1 0 0]
      settings: SourceProductName=IO691
  CAN pack : canmsglib/CAN Pack  MsgList=(none)  MsgName=enable  MsgIDType=Standard (11-bit identifier)  MsgIdentifier=id  MsgLength=8  Remote=off  ApplyMinMax=off  BusOutput=off  SignalInfo={ 'Motor postition 8-H', '0', '8', 'LE', 'unsigned', 'Standard', '0', '1', '0', '-Inf', 'Inf'; 'Motor position 8-L', '8', '8', 'LE', 'unsigned', 'Standard', '0', '1', '0', '-Inf', 'Inf'; 'Motor seed 8-H', '16', '8', 'LE', 'unsigned', 'Standard', '0', '1', '0', '-Inf', 'Inf'; 'Motor speed 4-L', '28', '4', 'LE', 'unsigned', 'Standard', '0', '1', '0', '-Inf', 'Inf'; 'KP 4-H', '24', '4', 'LE', 'unsigned', 'Standard', '0', '1', '0', '-Inf', 'Inf'; 'KP 8-L', '32', '8', 'LE', 'unsigned', 'Standard', '0', '1', '0', '-Inf', 'Inf'; 'KP 8-H', '40', '8', 'LE', 'unsigned', 'Standard', '0', '1', '0', '-Inf', 'Inf'; 'KD 4-L', '52', '4', 'LE', 'unsigned', 'Standard', '0', '1', '0', '-Inf', 'Inf'; 'Current 4-H', '48', '4', 'LE', 'unsigned', 'Standard', '0', '1', '0', '-Inf', 'Inf'; 'Current 8-L', '56', '8', 'LE', 'unsigned', 'Standard', '0', '1', '0', '-Inf', 'Inf' }
      settings: DataFormat=raw data
  Constant{,1..6} (7 alike) : Constant  Value=hex2dec('FF')  OutDataTypeStr=uint8  SampleTime=-1
  Constant7 : Constant  Value=hex2dec('FC')  OutDataTypeStr=uint8  SampleTime=-1
  Mux : Mux  Inputs=8
  wires:
  CAN pack/1 -> CAN Write Motor Mode/1
  Mux/1 -> CAN pack/1
  Constant7/1 -> Mux/8
  Constant4/1 -> Mux/5
  Constant1/1 -> Mux/2
  Constant5/1 -> Mux/6
  Constant3/1 -> Mux/4
  Constant2/1 -> Mux/3
  Constant/1 -> Mux/1
  Constant6/1 -> Mux/7

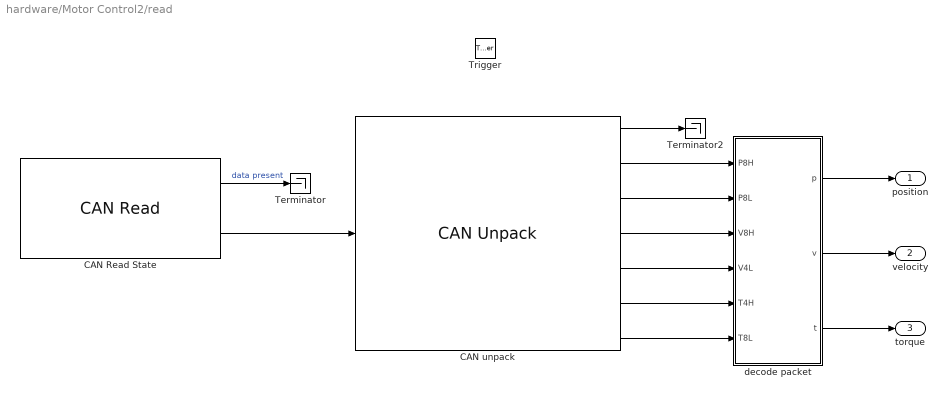
== system hardware/Motor Control2/read ==
  Trigger : TriggerPort  TriggerType=either  VariantControl=Variant
  CAN Read State : speedgoatlib_IO691/Legacy/CAN Read  id=1  ts=-1  channel=2  messageType=CAN  canType=CAN (HS)  BusOutput=off  initValues=[691 1 -1 1 1 1 0]
      settings: SourceProductName=IO691
  CAN unpack : canmsglib/CAN Unpack  MsgList=(none)  MsgName=CAN Msg  MsgIDType=Standard (11-bit identifier)  MsgIdentifier=0  MsgLength=6  SignalInfo={ 'ID', '0', '8', 'LE', 'unsigned', 'Standard', '0', '1', '0', '-Inf', 'Inf'; 'P8H', '8', '8', 'LE', 'unsigned', 'Standard', '0', '1', '0', '-Inf', 'Inf'; 'P8L', '16', '8', 'LE', 'unsigned', 'Standard', '0', '1', '0', '-Inf', 'Inf'; 'V8H', '24', '8', 'LE', 'unsigned', 'Standard', '0', '1', '0', '-Inf', 'Inf'; 'V4L', '36', '4', 'LE', 'unsigned', 'Standard', '0', '1', '0', '-Inf', 'Inf'; 'I4H', '32', '4', 'LE', 'unsigned', 'Standard', '0', '1', '0', '-Inf', 'Inf'; 'I8L', '40', '8', 'LE', 'unsigned', 'Standard', '0', '1', '0', '-Inf', 'Inf' }  IDPort=off  TimestampPort=off  ErrorPort=off  RemotePort=off  LengthPort=off  StatusPort=off  ApplyMinMax=off
  Terminator : Terminator
  Terminator2 : Terminator
  decode packet : MATLAB Function  TreatAsAtomicUnit=on
  position : Outport
  velocity : Outport  Port=2
  torque : Outport  Port=3
  wires:
  CAN unpack/1 -> Terminator2/1
  CAN Read State/2 -> CAN unpack/1
  CAN unpack/6 -> decode packet/5(T4H)
  CAN unpack/5 -> decode packet/4(V4L)
  CAN unpack/3 -> decode packet/2(P8L)
  CAN unpack/2 -> decode packet/1(P8H)
  CAN unpack/7 -> decode packet/6(T8L)
  CAN unpack/4 -> decode packet/3(V8H)
  decode packet/2(v) -> velocity/1
  decode packet/1(p) -> position/1
  decode packet/3(t) -> torque/1
  CAN Read State/1 -> Terminator/1  "data present"

== system hardware/Motor Control2/write ==
  pos_des : Inport
  vel_des : Inport  Port=2
  Kp : Inport  Port=3
  Kd : Inport  Port=4
  t_ff : Inport  Port=5
  Trigger : TriggerPort  VariantControl=Variant
  CAN Write Command : speedgoatlib_IO691/Legacy/CAN Write  id=1  ts=-1  channel=2  messageType=CAN  BusInput=off  enableStatusPort=off  canType=CAN (HS)  initValues=[691 1 -1 1 1 1 0 0]
      settings: SourceProductName=IO691
  CAN pack : canmsglib/CAN Pack  MsgList=(none)  MsgName=MotorControl  MsgIDType=Standard (11-bit identifier)  MsgIdentifier=id  MsgLength=8  Remote=off  ApplyMinMax=off  BusOutput=off  SignalInfo={ 'P8H', '0', '8', 'LE', 'unsigned', 'Standard', '0', '1', '0', '-Inf', 'Inf'; 'P8L', '8', '8', 'LE', 'unsigned', 'Standard', '0', '1', '0', '-Inf', 'Inf'; 'V8H', '16', '8', 'LE', 'unsigned', 'Standard', '0', '1', '0', '-Inf', 'Inf'; 'V4L', '28', '4', 'LE', 'unsigned', 'Standard', '0', '1', '0', '-Inf', 'Inf'; 'KP4H', '24', '4', 'LE', 'unsigned', 'Standard', '0', '1', '0', '-Inf', 'Inf'; 'KP8L', '32', '8', 'LE', 'unsigned', 'Standard', '0', '1', '0', '-Inf', 'Inf'; 'KD8H', '40', '8', 'LE', 'unsigned', 'Standard', '0', '1', '0', '-Inf', 'Inf'; 'KD4L', '52', '4', 'LE', 'unsigned', 'Standard', '0', '1', '0', '-Inf', 'Inf'; 'T4H', '48', '4', 'LE', 'unsigned', 'Standard', '0', '1', '0', '-Inf', 'Inf'; 'T8L', '56', '8', 'LE', 'unsigned', 'Standard', '0', '1', '0', '-Inf', 'Inf' }
      settings: DataFormat=manually specified signals
  encode packet : MATLAB Function  TreatAsAtomicUnit=on
  wires:
  vel_des/1 -> encode packet/2(v_des)
  pos_des/1 -> encode packet/1(p_des)
  encode packet/6(KP8L) -> CAN pack/6
  encode packet/7(KD8H) -> CAN pack/7
  encode packet/2(P8L) -> CAN pack/2
  Kp/1 -> encode packet/3(kp)
  encode packet/5(KP4H) -> CAN pack/5
  Kd/1 -> encode packet/4(kd)
  t_ff/1 -> encode packet/5(t_ff)
  encode packet/8(KD4L) -> CAN pack/8
  encode packet/4(V4L) -> CAN pack/4
  encode packet/9(T4H) -> CAN pack/9
  encode packet/1(P8H) -> CAN pack/1
  CAN pack/1 -> CAN Write Command/1
  encode packet/3(V8H) -> CAN pack/3
  encode packet/10(T8L) -> CAN pack/10

== matlab function hardware/Motor Control2/write/encode packet ==
  data: p_des input; P8H output; v_des input; kp input; kd input; t_ff input; P8L output; V8H output; V4L output; KP4H output; KP8L output; KD8H output; KD4L output; T4H output; T8L output
function [P8H,P8L,V8H,V4L,KP4H,KP8L,KD8H,KD4L,T4H,T8L] = encode(p_des, v_des, kp, kd, t_ff)
    % MOTOR CONSTANTS
    GR = 6; % Gear ratio
    KT = 0.28; % Torque Constant Nm/A
    P_MAX = 12.5; % rad
    P_MIN = -P_MAX; % rad
    V_MAX = 65.0; % rad/s
    V_MIN = -V_MAX; % rad/s
    I_MAX = 20.0; % A
    T_MAX = I_MAX*KT*GR; % Nm
    T_MIN = -I_MAX*KT*GR; % Nm
    KP_MAX = 500; % Nm/rad
    KP_MIN = 0; % Nm/rad
    KD_MAX = 5; % Nm/rad/s
    KD_MIN = 0; % Nm/rad/s
    % bound inputs
    p_des = min([max([P_MIN,p_des]),P_MAX]);
    v_des = min([max([V_MIN,v_des]),V_MAX]);
    kp = min([max([KP_MIN,kp]),KP_MAX]);
    kd = min([max([KD_MIN,kd]),KD_MAX]);
    t_ff = min([max([T_MIN,t_ff]),T_MAX]);
    
    % convert floats to unsigned integers
    p_int = float_to_uint(p_des, P_MIN, P_MAX, 16);
    v_int = float_to_uint(v_des, V_MIN, V_MAX, 12);
    kp_int = float_to_uint(kp, KP_MIN, KP_MAX, 12);
    kd_int = float_to_uint(kd, KD_MIN, KD_MAX, 12);
    t_int = float_to_uint(t_ff, T_MIN, T_MAX, 12);
    
    % break up for CAN frame 
    P8H = bitshift(p_int, -8); % 8 higher bits
    P8L = bitand(p_int, 0xFF); % 8 lower bits
    V8H = bitshift(v_int, -4); % 8 higher bits
    V4L = bitand(v_int, 0xF); % 4 lower bits
    KP4H = bitshift(kp_int, -8); % 4 higher bits
    KP8L = bitand(kp_int, 0xFF); % 8 lower bits
    KD8H = bitshift(kd_int, -4); % 8 higher bits
    KD4L = bitand(kd_int, 0xF); % 4 lower bits
    T4H = bitshift(t_int, -8); % 4 higher bits
    T8L = bitand(t_int, 0xFF); % 8 lower bits
    
    % Converts a float to an unsigned int, given range and number of bits
    function x_int = float_to_uint(x, x_min, x_max, n_bits)
        span = x_max - x_min;
        min([max([x_min,x]),x_max])
        x_int = ((x - x_min)*((bitshift(1, n_bits)-1) / span));
    end
end
%final_values = desired_pos,desired_vel,desired_kp,desired_kd,desired_tau;

== matlab function hardware/Motor Control1/write/encode packet ==
  data: p_des input; P8H output; v_des input; kp input; kd input; t_ff input; P8L output; V8H output; V4L output; KP4H output; KP8L output; KD8H output; KD4L output; T4H output; T8L output
function [P8H,P8L,V8H,V4L,KP4H,KP8L,KD8H,KD4L,T4H,T8L] = encode(p_des, v_des, kp, kd, t_ff)
    % MOTOR CONSTANTS
    GR = 6; % Gear ratio
    KT = 0.28; % Torque Constant Nm/A
    P_MAX = 12.5; % rad
    P_MIN = -P_MAX; % rad
    V_MAX = 65.0; % rad/s
    V_MIN = -V_MAX; % rad/s
    I_MAX = 20.0; % A
    T_MAX = I_MAX*KT*GR; % Nm
    T_MIN = -I_MAX*KT*GR; % Nm
    KP_MAX = 500; % Nm/rad
    KP_MIN = 0; % Nm/rad
    KD_MAX = 5; % Nm/rad/s
    KD_MIN = 0; % Nm/rad/s
    % bound inputs
    p_des = min([max([P_MIN,p_des]),P_MAX]);
    v_des = min([max([V_MIN,v_des]),V_MAX]);
    kp = min([max([KP_MIN,kp]),KP_MAX]);
    kd = min([max([KD_MIN,kd]),KD_MAX]);
    t_ff = min([max([T_MIN,t_ff]),T_MAX]);
    
    % convert floats to unsigned integers
    p_int = float_to_uint(p_des, P_MIN, P_MAX, 16);
    v_int = float_to_uint(v_des, V_MIN, V_MAX, 12);
    kp_int = float_to_uint(kp, KP_MIN, KP_MAX, 12);
    kd_int = float_to_uint(kd, KD_MIN, KD_MAX, 12);
    t_int = float_to_uint(t_ff, T_MIN, T_MAX, 12);
    
    % break up for CAN frame 
    P8H = bitshift(p_int, -8); % 8 higher bits
    P8L = bitand(p_int, 0xFF); % 8 lower bits
    V8H = bitshift(v_int, -4); % 8 higher bits
    V4L = bitand(v_int, 0xF); % 4 lower bits
    KP4H = bitshift(kp_int, -8); % 4 higher bits
    KP8L = bitand(kp_int, 0xFF); % 8 lower bits
    KD8H = bitshift(kd_int, -4); % 8 higher bits
    KD4L = bitand(kd_int, 0xF); % 4 lower bits
    T4H = bitshift(t_int, -8); % 4 higher bits
    T8L = bitand(t_int, 0xFF); % 8 lower bits
    
    % Converts a float to an unsigned int, given range and number of bits
    function x_int = float_to_uint(x, x_min, x_max, n_bits)
        span = x_max - x_min;
        min([max([x_min,x]),x_max])
        x_int = ((x - x_min)*((bitshift(1, n_bits)-1) / span));
    end
end
%final_values = desired_pos,desired_vel,desired_kp,desired_kd,desired_tau;

== matlab function hardware/Motor Control1/read/decode packet ==
  data: P8H input; p output; P8L input; V8H input; V4L input; T4H input; T8L input; v output; t output
function [p, v, t] = decode(P8H,P8L,V8H,V4L,T4H,T8L)
    % MOTOR CONSTANTS
    GR = 6; % Gear ratio
    KT = 0.28; % Torque Constant Nm/A
    P_MAX = 12.5; % rad
    P_MIN = -P_MAX; % rad
    V_MAX = 65.0; % rad/s
    V_MIN = -V_MAX; % rad/s
    I_MAX = 20.0; % A
    T_MAX = I_MAX*KT*GR; % Nm
    T_MIN = -I_MAX*KT*GR; % Nm
    KP_MAX = 500; % Nm/rad
    KP_MIN = 0; % Nm/rad
    KD_MAX = 5; % Nm/rad/s
    KD_MIN = 0; % Nm/rad/s    

    % combine data
    p_int = bitor(bitshift(P8H, 8), P8L);
    v_int = bitor(bitshift(V8H, 4), V4L);
    t_int = bitor(bitshift(T4H, 8), T8L);
    
    % convert uints to floats
    p = uint_to_float(p_int, P_MIN, P_MAX, 16);
    v = uint_to_float(v_int, V_MIN, V_MAX, 12);
    t = uint_to_float(t_int, T_MIN, T_MAX, 12);

    % Converts a float to an unsigned int, given range and number of bits
    function x_float = uint_to_float(x, x_min, x_max, n_bits)
        span = x_max - x_min;
        offset = x_min;
        x_float = x * span / (bitshift(1, n_bits)-1) + offset;
    end
end

== matlab function hardware/Motor Control2/read/decode packet ==
  data: P8H input; p output; P8L input; V8H input; V4L input; T4H input; T8L input; v output; t output
function [p, v, t] = decode(P8H,P8L,V8H,V4L,T4H,T8L)
    % MOTOR CONSTANTS
    GR = 6; % Gear ratio
    KT = 0.28; % Torque Constant Nm/A
    P_MAX = 12.5; % rad
    P_MIN = -P_MAX; % rad
    V_MAX = 65.0; % rad/s
    V_MIN = -V_MAX; % rad/s
    I_MAX = 20.0; % A
    T_MAX = I_MAX*KT*GR; % Nm
    T_MIN = -I_MAX*KT*GR; % Nm
    KP_MAX = 500; % Nm/rad
    KP_MIN = 0; % Nm/rad
    KD_MAX = 5; % Nm/rad/s
    KD_MIN = 0; % Nm/rad/s    

    % combine data
    p_int = bitor(bitshift(P8H, 8), P8L);
    v_int = bitor(bitshift(V8H, 4), V4L);
    t_int = bitor(bitshift(T4H, 8), T8L);
    
    % convert uints to floats
    p = uint_to_float(p_int, P_MIN, P_MAX, 16);
    v = uint_to_float(v_int, V_MIN, V_MAX, 12);
    t = uint_to_float(t_int, T_MIN, T_MAX, 12);

    % Converts a float to an unsigned int, given range and number of bits
    function x_float = uint_to_float(x, x_min, x_max, n_bits)
        span = x_max - x_min;
        offset = x_min;
        x_float = x * span / (bitshift(1, n_bits)-1) + offset;
    end
end

== matlab function hardware/Motor 4/CAN Read/MATLAB Function ==
  data: pos output; pos_H input; pos_L input; vel_H input; vel_L input; current_H input; current_L input; vel output; i output
function [pos, vel, i]= motorDataConversion(pos_H, pos_L, vel_H, vel_L, current_H, current_L)
    % Output vectors for the motors
    % persistent Motor1Data;
    % persistent Motor2Data;
    % persistent Motor3Data;
    % persistent Motor4Data;
    % if isempty(Motor1Data) % Initialize variables
    %     Motor1Data = [NaN, NaN, NaN];
    %     Motor2Data = [NaN, NaN, NaN];
    %     Motor3Data = [NaN, NaN, NaN];
    %     Motor4Data = [NaN, NaN, NaN];
    % end
    % Convert bit values to units (rad, rad/s, A)
    % ------------------------------------
    max_pos = 12.5; 
    min_pos = -12.5; 
    span_pos = max_pos - min_pos;
    offset_pos = max_pos;
    
    pos = bitshift(pos_H,8);
    combined_pos = bitor(pos,pos_L);
    
    pos = ((combined_pos*span_pos)/(2^16-1))-offset_pos;
    
    % final_pos = (range_pos*4*pi)/12.5; % Zubair's use - needs checking, as
    % why are we not trusting the encoder readings?
    % ------------------------------------
    max_vel = 50;
    min_vel = -50;
    span_vel = max_vel - min_vel;
    offset_vel = max_vel;
    vel = bitshift(vel_H,4);
    combined_vel = bitor(vel,vel_L);
    
    vel = ((combined_vel*span_vel)/(2^12-1))-offset_vel;
    
    % ------------------------------------
    max_i = 65;
    min_i = -65;
    span_i = max_i - min_i;
    offset_i = max_i;
    i = bitshift(current_H,8);
    combined_i = bitor(i,current_L);
    
    i = ((combined_i*span_i)/(2^12-1))-offset_i;
    
   % switch CAN_ID
   %     case 1
   %         Motor1Data = [pos, vel, final_i];
   %     case 2
   %         Motor2Data = [pos, vel, final_i];
   %     case 3
   %         Motor3Data = [pos, vel, final_i];
   %     case 4
   %         Motor4Data = [pos, vel, final_i];
   % end
   % % Update the output (MATLAB doesn't want outputs to be persistents)
   % MotorStates = [Motor1Data, Motor2Data, Motor3Data, Motor4Data];
end

== matlab function hardware/Motor 4/CAN Write/MATLAB Function ==
  data: p_des input; P8H output; v_des input; kp input; kd input; t_ff input; P8L output; V8H output; M2L output; KP4H output; KP8L output; KD8H output; KD4L output; T4H output; T8L output
function [P8H,P8L,V8H,M2L,KP4H,KP8L,KD8H,KD4L,T4H,T8L] = AK1090(p_des, v_des, kp, kd, t_ff)
    % Coppied from AK70-10 manual
    % NB: CONSTANTS FOR AK70-10
    p_min = -12.5; % rad
    p_max = +12.5; % rad
    v_min = -50.0; % rad/s
    v_max = +50.0; % rad/s
    t_min = -65.0; % Nm
    t_max = +65.0; % Nm
    kp_min = 0;
    kp_max = 500;
    kd_min = 0;
    kd_max = 5;
    
    % bound inputs
    p_des = min([max([p_min,p_des]),p_max]);
    v_des = min([max([v_min,v_des]),v_max]);
    kp = min([max([kp_min,kp]),kp_max]);
    kd = min([max([kd_min,kd]),kd_max]);
    t_ff = min([max([t_min,t_ff]),t_max]);
    
    % convert floats to unsigned integers
    p_int = float_to_uint(p_des, p_min, p_max, 16);
    v_int = float_to_uint(v_des, v_min, v_max, 12);
    kp_int = float_to_uint(kp, kp_min, kp_max, 12);
    kd_int = float_to_uint(kd, kd_min, kd_max, 12);
    t_int = float_to_uint(t_ff, t_min, t_max, 12);
    
    % break up for CAN frame 
    P8H = bitshift(p_int, -8); % 8 higher bits
    P8L = bitand(p_int, 0xFF); % 8 lower bits
    V8H = bitshift(v_int, -4); % 8 higher bits
    M2L = bitand(v_int, 0xF); % 4 lower bits
    KP4H = bitshift(kp_int, -8); % 4 higher bits
    KP8L = bitand(kp_int, 0xFF); % 8 lower bits
    KD8H = bitshift(kd_int, -4); % 8 higher bits
    KD4L = bitand(kd_int, 0xF); % 4 lower bits
    T4H = bitshift(t_int, -8); % 4 higher bits
    T8L = bitand(t_int, 0xFF); % 8 lower bits
    
    % Converts a float to an unsigned int, given range and number of bits
    function x_int = float_to_uint(x, x_min, x_max, n_bits)
        span = x_max - x_min;
        min([max([x_min,x]),x_max])
        x_int = ((x - x_min)*(bitshift(1, n_bits) / span));
    end
end
%final_values = desired_pos,desired_vel,desired_kp,desired_kd,desired_tau;
